simulink model "Opcode_Register"  (R2024b)
settings: Solver=VariableStepAuto  StartTime=0.0  StopTime=10.0  RelTol=1e-3
settings Model: Creator=HP  LastModifiedBy=HP

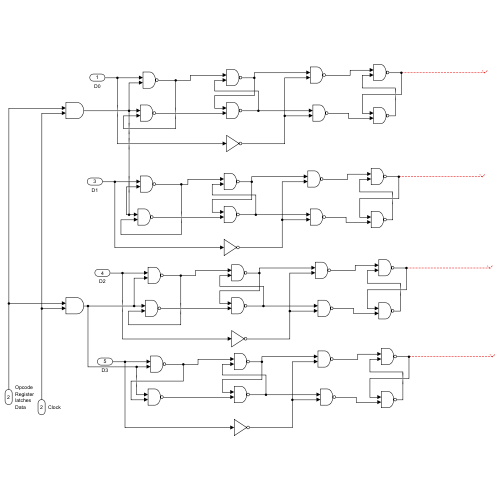
[thumbnail: Simulink's stored preview of the top-level diagram]
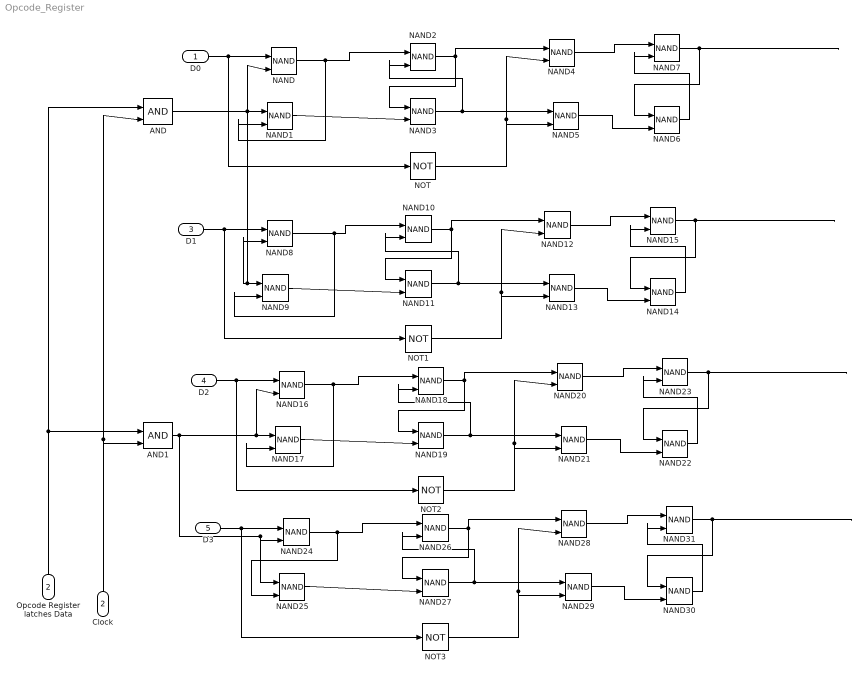
== system Opcode_Register ==
  D0 : Inport
  Opcode Register latches Data : Inport  Port=2
  D1 : Inport  Port=3
  D2 : Inport  Port=4
  D3 : Inport  Port=5
  AND : Logic  IconShape=distinctive  AllPortsSameDT=off  OutDataTypeStr=boolean
  AND1 : Logic  IconShape=distinctive  AllPortsSameDT=off  OutDataTypeStr=boolean
  Clock : InportShadow  Port=2
  NAND{,1..31} (32 alike) : Logic  Operator=NAND  IconShape=distinctive  AllPortsSameDT=off  OutDataTypeStr=boolean
  NOT{,1..3} (4 alike) : Logic  Operator=NOT  IconShape=distinctive  AllPortsSameDT=off  OutDataTypeStr=boolean
  wires:
  NAND/1 -> NAND1/2, NAND2/1
  NAND1/1 -> NAND3/2
  NAND2/1 -> NAND3/1, NAND4/1
  NAND3/1 -> NAND5/1, NAND2/2
  D0/1 -> NOT/1, NAND/1
  NOT/1 -> NAND5/2, NAND4/2
  NAND5/1 -> NAND6/2
  NAND4/1 -> NAND7/1
  NAND7/1 -> NAND6/1
  NAND6/1 -> NAND7/2
  Opcode Register latches Data/1 -> AND1/1, AND/1
  Clock/1 -> AND1/2, AND/2
  NAND9/1 -> NAND11/2
  NAND8/1 -> NAND9/2, NAND10/1
  D1/1 -> NOT1/1, NAND8/1
  NAND11/1 -> NAND13/1, NAND10/2
  NAND14/1 -> NAND15/2
  NAND15/1 -> NAND14/1
  NOT1/1 -> NAND13/2, NAND12/2
  NAND13/1 -> NAND14/2
  NAND10/1 -> NAND11/1, NAND12/1
  NAND12/1 -> NAND15/1
  AND/1 -> NAND8/2, NAND9/1, NAND1/1, NAND/2
  NAND17/1 -> NAND19/2
  NAND16/1 -> NAND17/2, NAND18/1
  D2/1 -> NOT2/1, NAND16/1
  NAND19/1 -> NAND21/1, NAND18/2
  NAND22/1 -> NAND23/2
  NAND23/1 -> NAND22/1
  NOT2/1 -> NAND21/2, NAND20/2
  NAND21/1 -> NAND22/2
  NAND18/1 -> NAND20/1, NAND19/1
  NAND20/1 -> NAND23/1
  NAND25/1 -> NAND27/2
  NAND24/1 -> NAND25/2, NAND26/1
  D3/1 -> NOT3/1, NAND24/1
  NAND27/1 -> NAND29/1, NAND26/2
  NAND30/1 -> NAND31/2
  NAND31/1 -> NAND30/1
  NOT3/1 -> NAND29/2, NAND28/2
  NAND29/1 -> NAND30/2
  NAND26/1 -> NAND27/1, NAND28/1
  NAND28/1 -> NAND31/1
  AND1/1 -> NAND17/1, NAND16/2, NAND25/1, NAND24/2
